simulink model "gm_LLE"  (R2020a)
settings: Solver=FixedStepDiscrete  StartTime=0.0  StopTime=T  FixedStep=1  RelTol=1e-3
InitFcn:
  | img_path = get_param('LLE/LowLightImage','FileName');
  | img = imread(img_path);
  | [m,n,c] = size(img);
  | 
  | h = [1, 2, 1; 2, 4, 2; 1, 2 ,1]./16;
  | h1 = flipud(fliplr(h));
  | T = (4000+(m+20)*(n+20));
undefined symbols (not defined in the file or in its folder): gray, m, n
libraries: visionfilter x10, visionhdlfilter x5, visionhdlio x4, visionhdlutilities x1, visionsources x1
settings Model: SimulationMode=accelerator  Creator=The MathWorks, Inc.  LastModifiedBy=25503
settings DataIOCC: ReturnWorkspaceOutputs=off
settings OptimizationCC: BlockReduction=off  ConditionallyExecuteInputs=off  DefaultParameterBehavior=Inlined
settings DebuggingCC: AlgebraicLoopMsg=error  InheritedTsInSrcMsg=none  ParameterPrecisionLossMsg=none  ArithmeticOperatorsInVariantConditions=warning
settings HardwareCC: ProdBitPerPointer=32  ProdBitPerSizeT=32  ProdBitPerPtrDiffT=32  ProdLargestAtomicFloat=None  ProdIntDivRoundTo=Undefined  ProdEndianess=Unspecified  ProdWordSize=32  ProdHWDeviceType=ASIC/FPGA->ASIC/FPGA  TargetBitPerPointer=64  TargetBitPerSizeT=64  TargetBitPerPtrDiffT=64  TargetLongLongMode=on  TargetIntDivRoundTo=Zero  TargetEndianess=LittleEndian  TargetWordSize=64  TargetHWDeviceType=Custom Processor->MATLAB Host Computer  ProdEqTarget=off
settings SFSimCC: SimUseLocalCustomCode=off  CustomCodeUndefinedFunction=UseInterfaceOnly
settings RTWCC: RTWUseLocalCustomCode=off

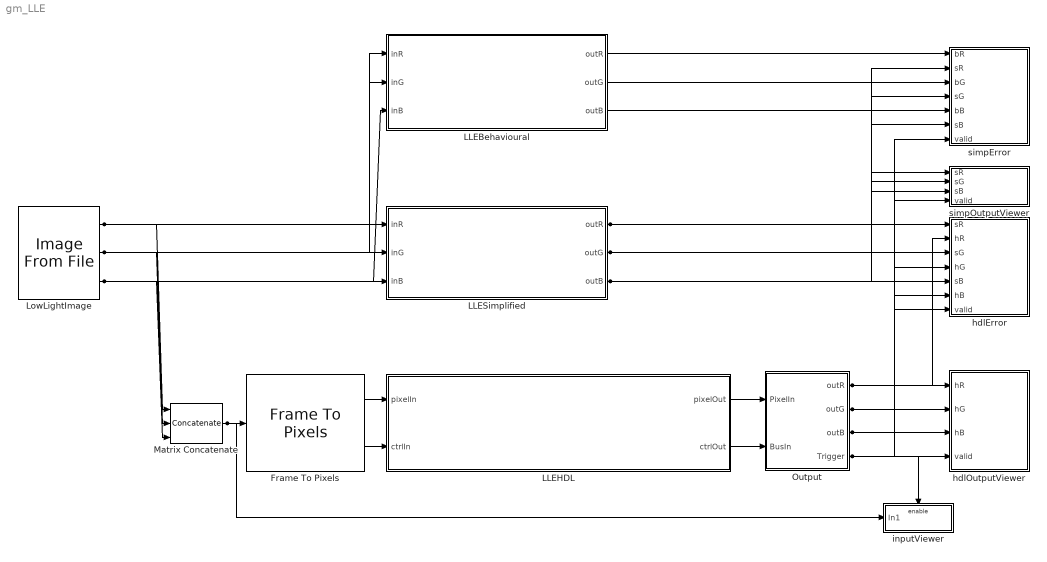
== system gm_LLE ==
  Frame To Pixels : visionhdlio/Frame To Pixels  NumComponents=c  NumPixels=1  VideoFormat=Custom  ActivePixelsPerLine=n  ActiveVideoLines=m  TotalPixelsPerLine=n+20  TotalVideoLines=m+20  StartingActiveLine=11  FrontPorch=10  SampleTime=0
      settings: SourceProductBaseCode=VT
  LLEBehavioural : Subsystem
  LLEHDL : Subsystem
  LLESimplified : Subsystem
  LowLightImage : visionsources/Image From File  Tag=vipblks_nd  FileName=C:\signal2\LLEHDL\myinput.jpg  Ts=(m+20)*(n+20)  imagePorts=Separate color signals  OutPortLabels=R|G|B  ImageDataType=Inherit from input image  sdImageDataType=uint(8)  Signed=on  WordLength=16  FractionLengthMode=User-defined  FractionLength=15
  Matrix Concatenate : Concatenate  NumInputs=3  Mode=Multidimensional array  ConcatenateDimension=3
  Output : Subsystem
  hdlError : Subsystem
  hdlOutputViewer : Subsystem
  inputViewer : Subsystem
  simpError : Subsystem
  simpOutputViewer : Subsystem
  wires:
  LLEBehavioural/2(outG) -> simpError/3(bG)
  LLEBehavioural/3(outB) -> simpError/5(bB)
  LLEBehavioural/1(outR) -> simpError/1(bR)
  LLESimplified/1(outR) -> hdlError/1(sR), simpOutputViewer/1(sR), simpError/2(sR)
  Matrix Concatenate/1 -> inputViewer/1(In1), Frame To Pixels/1
  Output/4(Trigger) -> inputViewer/Enable, hdlError/7(valid), simpOutputViewer/4(valid), simpError/7(valid), hdlOutputViewer/4(valid)
  LLESimplified/3(outB) -> hdlError/5(sB), simpOutputViewer/3(sB), simpError/6(sB)
  LLESimplified/2(outG) -> hdlError/3(sG), simpOutputViewer/2(sG), simpError/4(sG)
  Output/2(outG) -> hdlOutputViewer/2(hG), hdlError/4(hG)
  Output/1(outR) -> hdlError/2(hR), hdlOutputViewer/1(hR)
  Output/3(outB) -> hdlOutputViewer/3(hB), hdlError/6(hB)
  LowLightImage/3 -> Matrix Concatenate/3, LLEBehavioural/3(inB), LLESimplified/3(inB)
  LowLightImage/2 -> Matrix Concatenate/2, LLESimplified/2(inG), LLEBehavioural/2(inG)
  LowLightImage/1 -> Matrix Concatenate/1, LLEBehavioural/1(inR), LLESimplified/1(inR)
  LLEHDL/2(ctrlOut) -> Output/2(BusIn)
  LLEHDL/1(pixelOut) -> Output/1(PixelIn)
  Frame To Pixels/2 -> LLEHDL/2(ctrlIn)
  Frame To Pixels/1 -> LLEHDL/1(pixelIn)

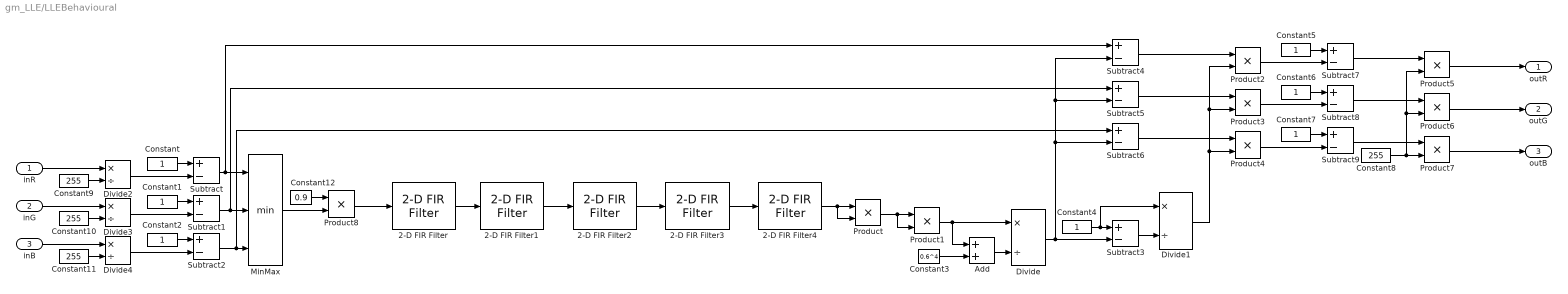
== system gm_LLE/LLEBehavioural ==
  inR : Inport
  inG : Inport  Port=2
  inB : Inport  Port=3
  2-D FIR Filter{,1..4} (5 alike) : visionfilter/2-D FIR Filter  separable=off  filtSrc=Specify via dialog  filterMtrx=h  verticalFilter=[4 0]  horizontalFilter=[4 0]  outSize=Same as input port I  padType=Replicate  padSrc=Specify via dialog  padVal=0  method=Convolution  firstCoeffMode=Binary point scaling  firstCoeffWordLength=16  firstCoeffFracLength=0  firstCoeffSignedness=Signed  firstCoeffLastDataTypeStr=fixdt(1,16,0)  outputSignedness=Auto  accumLastDataTypeStr=Inherit: Same as product output  roundingMode=Floor  overflowMode=off  firstCoeffDataTypeStr=fixdt(1,16,0)  firstCoeffMin=[]  firstCoeffMax=[]  accumDataTypeStr=Inherit: Same as product output  outputMin=[]  outputMax=[]
      settings: SourceProductBaseCode=VP
  Add : Sum
  Constant{,1..2,4..7} (7 alike) : Constant
  Constant10 : Constant  Value=255  OutDataTypeStr=double
  Constant11 : Constant  Value=255  OutDataTypeStr=double
  Constant12 : Constant  Value=0.9
  Constant3 : Constant  Value=0.6^4
  Constant8 : Constant  Value=255  OutDataTypeStr=uint8
  Constant9 : Constant  Value=255  OutDataTypeStr=double
  Divide{,1..4} (5 alike) : Product  Inputs=*/
  MinMax : MinMax  Inputs=3
  Product{,1..4,8} (6 alike) : Product
  Product5 : Product  OutDataTypeStr=uint8  RndMeth=Nearest  SaturateOnIntegerOverflow=on
  Product6 : Product  OutDataTypeStr=uint8  RndMeth=Nearest  SaturateOnIntegerOverflow=on
  Product7 : Product  OutDataTypeStr=uint8  RndMeth=Nearest  SaturateOnIntegerOverflow=on
  Subtract{,1..9} (10 alike) : Sum  Inputs=+-
  outR : Outport  VectorParamsAs1DForOutWhenUnconnected=off
  outG : Outport  Port=2  VectorParamsAs1DForOutWhenUnconnected=off
  outB : Outport  Port=3  VectorParamsAs1DForOutWhenUnconnected=off
  wires:
  Product7/1 -> outB/1
  inB/1 -> Divide4/1
  inG/1 -> Divide3/1
  Subtract5/1 -> Product3/1
  Constant12/1 -> Product8/1
  2-D FIR Filter3/1 -> 2-D FIR Filter4/1
  Constant5/1 -> Subtract7/1
  Product8/1 -> 2-D FIR Filter/1
  Constant6/1 -> Subtract8/1
  MinMax/1 -> Product8/2
  Subtract4/1 -> Product2/1
  Subtract9/1 -> Product7/1
  Product2/1 -> Subtract7/2
  Constant2/1 -> Subtract2/1
  Subtract8/1 -> Product6/1
  Constant8/1 -> Product5/2, Product6/2, Product7/2
  Product1/1 -> Divide/1, Add/1
  Subtract3/1 -> Divide1/2
  Product4/1 -> Subtract9/2
  Subtract2/1 -> MinMax/3, Subtract6/1
  Product6/1 -> outG/1
  Constant3/1 -> Add/2
  inR/1 -> Divide2/1
  Subtract6/1 -> Product4/1
  2-D FIR Filter1/1 -> 2-D FIR Filter2/1
  Subtract1/1 -> MinMax/2, Subtract5/1
  Constant4/1 -> Subtract3/1, Divide1/1
  Subtract7/1 -> Product5/1
  Product3/1 -> Subtract8/2
  Constant10/1 -> Divide3/2
  2-D FIR Filter/1 -> 2-D FIR Filter1/1
  2-D FIR Filter2/1 -> 2-D FIR Filter3/1
  Constant9/1 -> Divide2/2
  Subtract/1 -> MinMax/1, Subtract4/1
  Divide3/1 -> Subtract1/2
  Constant1/1 -> Subtract1/1
  Constant7/1 -> Subtract9/1
  Divide1/1 -> Product3/2, Product2/2, Product4/2
  Divide/1 -> Subtract3/2, Subtract6/2, Subtract4/2, Subtract5/2
  Constant11/1 -> Divide4/2
  Constant/1 -> Subtract/1
  Product/1 -> Product1/1, Product1/2
  Divide2/1 -> Subtract/2
  2-D FIR Filter4/1 -> Product/1, Product/2
  Divide4/1 -> Subtract2/2
  Add/1 -> Divide/2
  Product5/1 -> outR/1

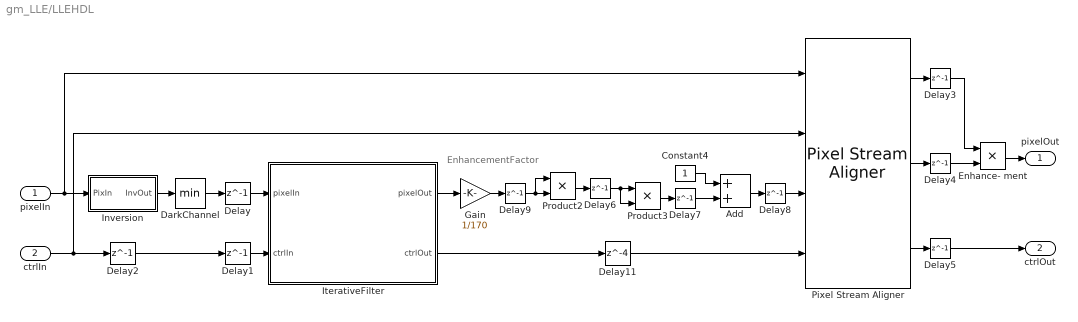
== system gm_LLE/LLEHDL ==
  note: EnhancementFactor
  pixelIn : Inport
  ctrlIn : Inport  Port=2
  Add : Sum  OutDataTypeStr=fixdt(0,30,22)  RndMeth=Nearest  SaturateOnIntegerOverflow=on
  Constant4 : Constant  OutDataTypeStr=fixdt(0,8,0)  SampleTime=-1
  DarkChannel : MinMax  RndMeth=Nearest  SaturateOnIntegerOverflow=on
  Delay{,1..9} (10 alike) : Delay  DelayLength=1
  Delay11 : Delay  DelayLength=4
  Enhance- ment : Product  OutDataTypeStr=uint8  RndMeth=Nearest  SaturateOnIntegerOverflow=on
  Gain : Gain  Gain=1/170  ParamDataTypeStr=fixdt(0,24,20)  OutDataTypeStr=fixdt(0,24,22)
  Inversion : Subsystem
  IterativeFilter : Subsystem
  Pixel Stream Aligner : visionhdlutilities/Pixel Stream Aligner  LineBufferSize=n  MaximumNumberOfLines=6  SimulateUsing=Code generation
      settings: SourceProductBaseCode=VT
  Product2 : Product  OutDataTypeStr=fixdt(0,26,22)  RndMeth=Nearest  SaturateOnIntegerOverflow=on
  Product3 : Product  OutDataTypeStr=fixdt(0,30,22)  RndMeth=Nearest  SaturateOnIntegerOverflow=on
  pixelOut : Outport  VectorParamsAs1DForOutWhenUnconnected=off
  ctrlOut : Outport  Port=2  VectorParamsAs1DForOutWhenUnconnected=off
  wires:
  IterativeFilter/2(ctrlOut) -> Delay11/1
  Delay9/1 -> Product2/2, Product2/1
  Delay5/1 -> ctrlOut/1
  Enhance- ment/1 -> pixelOut/1
  Delay11/1 -> Pixel Stream Aligner/4
  Delay8/1 -> Pixel Stream Aligner/3
  Gain/1 -> Delay9/1
  Delay/1 -> IterativeFilter/1(pixelIn)
  Delay1/1 -> IterativeFilter/2(ctrlIn)
  Add/1 -> Delay8/1
  Delay7/1 -> Add/2
  Delay6/1 -> Product3/1, Product3/2
  Constant4/1 -> Add/1
  Product3/1 -> Delay7/1
  Product2/1 -> Delay6/1
  IterativeFilter/1(pixelOut) -> Gain/1
  ctrlIn/1 -> Pixel Stream Aligner/2, Delay2/1
  Inversion/1(InvOut) -> DarkChannel/1
  Delay4/1 -> Enhance- ment/2
  Delay3/1 -> Enhance- ment/1
  Delay2/1 -> Delay1/1
  DarkChannel/1 -> Delay/1
  Pixel Stream Aligner/2 -> Delay4/1
  pixelIn/1 -> Pixel Stream Aligner/1, Inversion/1(PixIn)
  Pixel Stream Aligner/3 -> Delay5/1
  Pixel Stream Aligner/1 -> Delay3/1

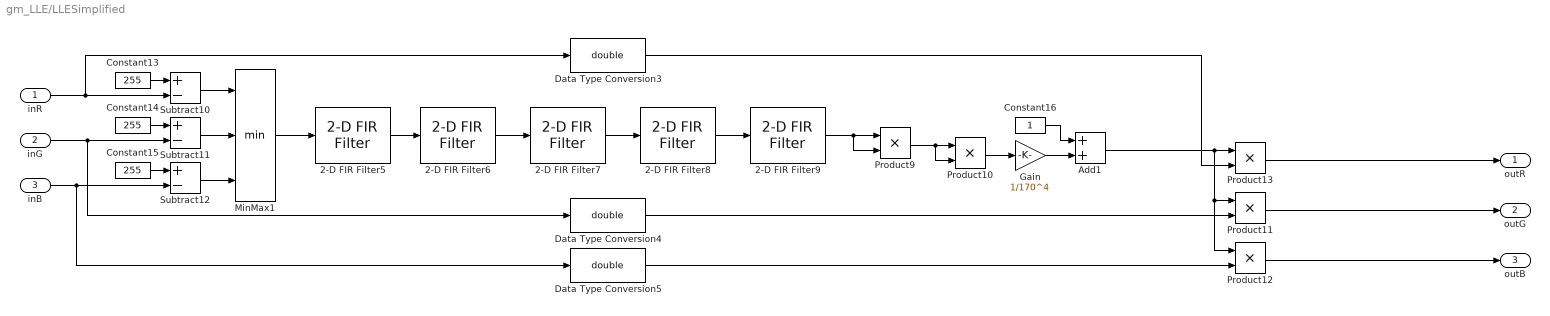
== system gm_LLE/LLESimplified ==
  inR : Inport
  inG : Inport  Port=2
  inB : Inport  Port=3
  2-D FIR Filter{5..9} (5 alike) : visionfilter/2-D FIR Filter  separable=off  filtSrc=Specify via dialog  filterMtrx=h  verticalFilter=[4 0]  horizontalFilter=[4 0]  outSize=Same as input port I  padType=Replicate  padSrc=Specify via dialog  padVal=0  method=Convolution  firstCoeffMode=Binary point scaling  firstCoeffWordLength=16  firstCoeffFracLength=0  firstCoeffSignedness=Signed  firstCoeffLastDataTypeStr=fixdt(1,16,0)  outputSignedness=Auto  accumLastDataTypeStr=Inherit: Same as product output  roundingMode=Floor  overflowMode=off  firstCoeffDataTypeStr=fixdt(1,16,0)  firstCoeffMin=[]  firstCoeffMax=[]  accumDataTypeStr=Inherit: Same as product output  outputMin=[]  outputMax=[]
      settings: SourceProductBaseCode=VP
  Add1 : Sum
  Constant13 : Constant  Value=255
  Constant14 : Constant  Value=255
  Constant15 : Constant  Value=255
  Constant16 : Constant
  Data Type Conversion3 : DataTypeConversion  OutDataTypeStr=double
  Data Type Conversion4 : DataTypeConversion  OutDataTypeStr=double
  Data Type Conversion5 : DataTypeConversion  OutDataTypeStr=double
  Gain : Gain  Gain=1/170^4
  MinMax1 : MinMax  Inputs=3
  Product10 : Product
  Product11 : Product  OutDataTypeStr=uint8  RndMeth=Nearest  SaturateOnIntegerOverflow=on
  Product12 : Product  OutDataTypeStr=uint8  RndMeth=Nearest  SaturateOnIntegerOverflow=on
  Product13 : Product  OutDataTypeStr=uint8  RndMeth=Nearest  SaturateOnIntegerOverflow=on
  Product9 : Product
  Subtract10 : Sum  Inputs=+-
  Subtract11 : Sum  Inputs=+-
  Subtract12 : Sum  Inputs=+-
  outR : Outport  VectorParamsAs1DForOutWhenUnconnected=off
  outG : Outport  Port=2  VectorParamsAs1DForOutWhenUnconnected=off
  outB : Outport  Port=3  VectorParamsAs1DForOutWhenUnconnected=off
  wires:
  Data Type Conversion5/1 -> Product12/2
  Data Type Conversion4/1 -> Product11/2
  Data Type Conversion3/1 -> Product13/2
  Product11/1 -> outG/1
  Product13/1 -> outR/1
  Constant13/1 -> Subtract10/1
  Constant16/1 -> Add1/1
  2-D FIR Filter9/1 -> Product9/2, Product9/1
  Constant14/1 -> Subtract11/1
  MinMax1/1 -> 2-D FIR Filter5/1
  Subtract10/1 -> MinMax1/1
  Add1/1 -> Product13/1, Product11/1, Product12/1
  2-D FIR Filter7/1 -> 2-D FIR Filter8/1
  2-D FIR Filter5/1 -> 2-D FIR Filter6/1
  Product9/1 -> Product10/1, Product10/2
  2-D FIR Filter6/1 -> 2-D FIR Filter7/1
  Product10/1 -> Gain/1
  inB/1 -> Subtract12/2, Data Type Conversion5/1
  Subtract12/1 -> MinMax1/3
  Gain/1 -> Add1/2
  inR/1 -> Subtract10/2, Data Type Conversion3/1
  Subtract11/1 -> MinMax1/2
  2-D FIR Filter8/1 -> 2-D FIR Filter9/1
  Product12/1 -> outB/1
  inG/1 -> Subtract11/2, Data Type Conversion4/1
  Constant15/1 -> Subtract12/1

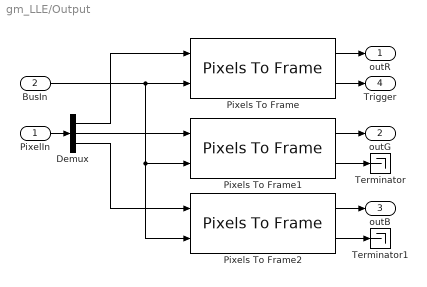
== system gm_LLE/Output ==
  PixelIn : Inport
  BusIn : Inport  Port=2
  Demux : Demux  Outputs=3
  Pixels To Frame : visionhdlio/Pixels To Frame  NumComponents=1  NumPixels=1  VideoFormat=Custom  ActivePixelsPerLine=n  ActiveVideoLines=m  TotalPixelsPerLine=n+20  TotalVideoLines=m+20
      settings: SourceProductBaseCode=VT
  Pixels To Frame1 : visionhdlio/Pixels To Frame  NumComponents=1  NumPixels=1  VideoFormat=Custom  ActivePixelsPerLine=n  ActiveVideoLines=m  TotalPixelsPerLine=n+20  TotalVideoLines=m+20
      settings: SourceProductBaseCode=VT
  Pixels To Frame2 : visionhdlio/Pixels To Frame  NumComponents=1  NumPixels=1  VideoFormat=Custom  ActivePixelsPerLine=n  ActiveVideoLines=m  TotalPixelsPerLine=n+20  TotalVideoLines=m+20
      settings: SourceProductBaseCode=VT
  Terminator : Terminator
  Terminator1 : Terminator
  outR : Outport  VectorParamsAs1DForOutWhenUnconnected=off
  outG : Outport  Port=2  VectorParamsAs1DForOutWhenUnconnected=off
  outB : Outport  Port=3  VectorParamsAs1DForOutWhenUnconnected=off
  Trigger : Outport  Port=4  VectorParamsAs1DForOutWhenUnconnected=off
  wires:
  Demux/1 -> Pixels To Frame/1
  PixelIn/1 -> Demux/1
  Pixels To Frame2/2 -> Terminator1/1
  BusIn/1 -> Pixels To Frame/2, Pixels To Frame1/2, Pixels To Frame2/2
  Demux/3 -> Pixels To Frame2/1
  Pixels To Frame2/1 -> outB/1
  Pixels To Frame1/2 -> Terminator/1
  Demux/2 -> Pixels To Frame1/1
  Pixels To Frame1/1 -> outG/1
  Pixels To Frame/2 -> Trigger/1
  Pixels To Frame/1 -> outR/1

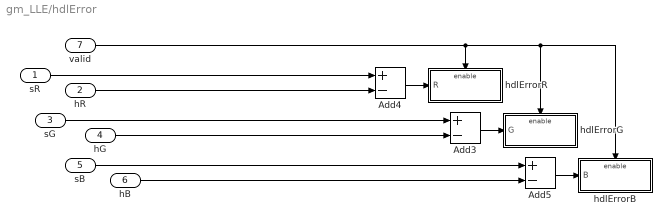
== system gm_LLE/hdlError ==
  sR : Inport
  hR : Inport  Port=2
  sG : Inport  Port=3
  hG : Inport  Port=4
  sB : Inport  Port=5
  hB : Inport  Port=6
  valid : Inport  Port=7
  Add3 : Sum  Inputs=+-  OutDataTypeStr=uint8  RndMeth=Nearest
  Add4 : Sum  Inputs=+-  OutDataTypeStr=uint8  RndMeth=Nearest
  Add5 : Sum  Inputs=+-  OutDataTypeStr=uint8  RndMeth=Nearest
  hdlErrorB : Subsystem
  hdlErrorG : Subsystem
  hdlErrorR : Subsystem
  wires:
  sR/1 -> Add4/1
  sB/1 -> Add5/1
  valid/1 -> hdlErrorR/Enable, hdlErrorG/Enable, hdlErrorB/Enable
  hG/1 -> Add3/2
  hR/1 -> Add4/2
  hB/1 -> Add5/2
  sG/1 -> Add3/1
  Add3/1 -> hdlErrorG/1(G)
  Add5/1 -> hdlErrorB/1(B)
  Add4/1 -> hdlErrorR/1(R)

== system gm_LLE/hdlOutputViewer ==
  hR : Inport
  hG : Inport  Port=2
  hB : Inport  Port=3
  valid : Inport  Port=4
  Matrix Concatenate1 : Concatenate  NumInputs=3  Mode=Multidimensional array  ConcatenateDimension=3
  hdlOutputViewer : Subsystem
  wires:
  valid/1 -> hdlOutputViewer/Enable
  hR/1 -> Matrix Concatenate1/1
  hB/1 -> Matrix Concatenate1/3
  hG/1 -> Matrix Concatenate1/2
  Matrix Concatenate1/1 -> hdlOutputViewer/1(In1)

== system gm_LLE/inputViewer ==
  In1 : Inport
  Enable : EnablePort
  LLEInput : VideoViewer  colormapValue=gray(256)  FigPos=[55.4 550.8 353.6 289.6]
  wires:
  In1/1 -> LLEInput/1

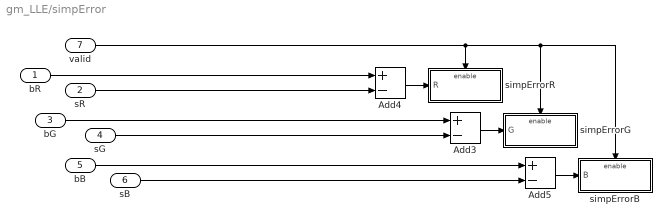
== system gm_LLE/simpError ==
  bR : Inport
  sR : Inport  Port=2
  bG : Inport  Port=3
  sG : Inport  Port=4
  bB : Inport  Port=5
  sB : Inport  Port=6
  valid : Inport  Port=7
  Add3 : Sum  Inputs=+-  OutDataTypeStr=uint8  RndMeth=Nearest
  Add4 : Sum  Inputs=+-  OutDataTypeStr=uint8  RndMeth=Nearest
  Add5 : Sum  Inputs=+-  OutDataTypeStr=uint8  RndMeth=Nearest
  simpErrorB : Subsystem
  simpErrorG : Subsystem
  simpErrorR : Subsystem
  wires:
  bR/1 -> Add4/1
  bB/1 -> Add5/1
  valid/1 -> simpErrorR/Enable, simpErrorG/Enable, simpErrorB/Enable
  sG/1 -> Add3/2
  sR/1 -> Add4/2
  sB/1 -> Add5/2
  bG/1 -> Add3/1
  Add3/1 -> simpErrorG/1(G)
  Add5/1 -> simpErrorB/1(B)
  Add4/1 -> simpErrorR/1(R)

== system gm_LLE/simpOutputViewer ==
  sR : Inport
  sG : Inport  Port=2
  sB : Inport  Port=3
  valid : Inport  Port=4
  Matrix Concatenate1 : Concatenate  NumInputs=3  Mode=Multidimensional array  ConcatenateDimension=3
  simpOutputViewer : Subsystem
  wires:
  valid/1 -> simpOutputViewer/Enable
  sR/1 -> Matrix Concatenate1/1
  sB/1 -> Matrix Concatenate1/3
  sG/1 -> Matrix Concatenate1/2
  Matrix Concatenate1/1 -> simpOutputViewer/1(In1)

== system gm_LLE/LLEHDL/Inversion ==
  PixIn : Inport
  Constant : Constant  Value=255  OutDataTypeStr=fixdt(0,8,0)  SampleTime=-1
  Delay : Delay  DelayLength=1
  Subtract : Sum  Inputs=+-  OutDataTypeStr=uint8  RndMeth=Nearest  SaturateOnIntegerOverflow=on
  InvOut : Outport  VectorParamsAs1DForOutWhenUnconnected=off
  wires:
  Delay/1 -> InvOut/1
  PixIn/1 -> Subtract/2
  Subtract/1 -> Delay/1
  Constant/1 -> Subtract/1

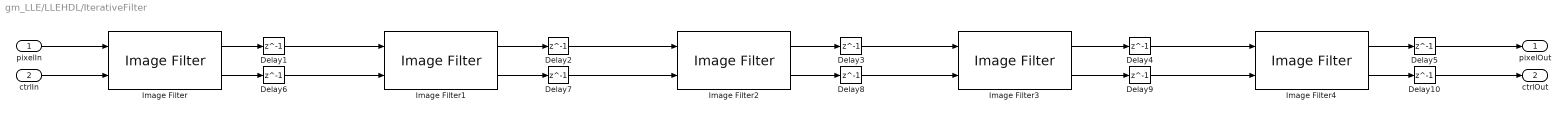
== system gm_LLE/LLEHDL/IterativeFilter ==
  pixelIn : Inport
  ctrlIn : Inport  Port=2
  Delay{1..10} (10 alike) : Delay  DelayLength=1
  Image Filter : visionhdlfilter/Image Filter  CoefficientsSource=Property  Coefficients=h1  PaddingMethod=Replicate  PaddingValue=0  LineBufferSize=2*n  SimulateUsing=Code generation  roundingMode=Nearest  overflowMode=on  CoeffDataTypeStr=fixdt(0,4,4)  CoeffMin=[]  CoeffMax=[]  OutputDataTypeStr=fixdt(0,12,4)  OutputMin=[]  OutputMax=[]
      settings: SourceProductBaseCode=VT
  Image Filter1 : visionhdlfilter/Image Filter  CoefficientsSource=Property  Coefficients=h1  PaddingMethod=Replicate  PaddingValue=0  LineBufferSize=2*n  SimulateUsing=Code generation  roundingMode=Nearest  overflowMode=on  CoeffDataTypeStr=fixdt(0,4,4)  CoeffMin=[]  CoeffMax=[]  OutputDataTypeStr=fixdt(0,16,8)  OutputMin=[]  OutputMax=[]
      settings: SourceProductBaseCode=VT
  Image Filter2 : visionhdlfilter/Image Filter  CoefficientsSource=Property  Coefficients=h1  PaddingMethod=Replicate  PaddingValue=0  LineBufferSize=2*n  SimulateUsing=Code generation  roundingMode=Nearest  overflowMode=on  CoeffDataTypeStr=fixdt(0,4,4)  CoeffMin=[]  CoeffMax=[]  OutputDataTypeStr=fixdt(0,20,12)  OutputMin=[]  OutputMax=[]
      settings: SourceProductBaseCode=VT
  Image Filter3 : visionhdlfilter/Image Filter  CoefficientsSource=Property  Coefficients=h1  PaddingMethod=Replicate  PaddingValue=0  LineBufferSize=2*n  SimulateUsing=Code generation  roundingMode=Nearest  overflowMode=on  CoeffDataTypeStr=fixdt(0,4,4)  CoeffMin=[]  CoeffMax=[]  OutputDataTypeStr=fixdt(0,24,16)  OutputMin=[]  OutputMax=[]
      settings: SourceProductBaseCode=VT
  Image Filter4 : visionhdlfilter/Image Filter  CoefficientsSource=Property  Coefficients=h1  PaddingMethod=Replicate  PaddingValue=0  LineBufferSize=2*n  SimulateUsing=Code generation  roundingMode=Nearest  overflowMode=on  CoeffDataTypeStr=fixdt(0,4,4)  CoeffMin=[]  CoeffMax=[]  OutputDataTypeStr=fixdt(0,28,20)  OutputMin=[]  OutputMax=[]
      settings: SourceProductBaseCode=VT
  pixelOut : Outport  VectorParamsAs1DForOutWhenUnconnected=off
  ctrlOut : Outport  Port=2  VectorParamsAs1DForOutWhenUnconnected=off
  wires:
  Delay10/1 -> ctrlOut/1
  Delay5/1 -> pixelOut/1
  Delay4/1 -> Image Filter4/1
  Delay9/1 -> Image Filter4/2
  Delay8/1 -> Image Filter3/2
  Delay3/1 -> Image Filter3/1
  Delay2/1 -> Image Filter2/1
  Delay7/1 -> Image Filter2/2
  Delay6/1 -> Image Filter1/2
  Delay1/1 -> Image Filter1/1
  Image Filter4/2 -> Delay10/1
  Image Filter4/1 -> Delay5/1
  Image Filter3/1 -> Delay4/1
  Image Filter2/1 -> Delay3/1
  Image Filter1/1 -> Delay2/1
  Image Filter/1 -> Delay1/1
  ctrlIn/1 -> Image Filter/2
  pixelIn/1 -> Image Filter/1
  Image Filter/2 -> Delay6/1
  Image Filter1/2 -> Delay7/1
  Image Filter2/2 -> Delay8/1
  Image Filter3/2 -> Delay9/1

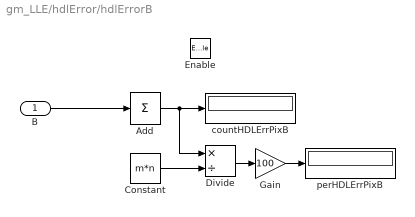
== system gm_LLE/hdlError/hdlErrorB ==
  B : Inport
  Enable : EnablePort
  Add : Sum  Inputs=+
  Constant : Constant  Value=m*n
  Divide : Product  Inputs=*/
  Gain : Gain  Gain=100
  countHDLErrPixB : Display
  perHDLErrPixB : Display
  wires:
  Divide/1 -> Gain/1
  Add/1 -> countHDLErrPixB/1, Divide/1
  Constant/1 -> Divide/2
  Gain/1 -> perHDLErrPixB/1
  B/1 -> Add/1

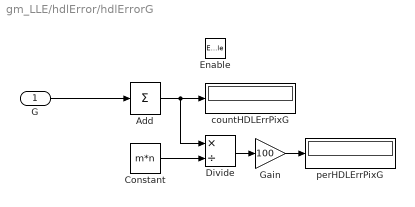
== system gm_LLE/hdlError/hdlErrorG ==
  G : Inport
  Enable : EnablePort
  Add : Sum  Inputs=+
  Constant : Constant  Value=m*n
  Divide : Product  Inputs=*/
  Gain : Gain  Gain=100
  countHDLErrPixG : Display
  perHDLErrPixG : Display
  wires:
  Gain/1 -> perHDLErrPixG/1
  Constant/1 -> Divide/2
  Add/1 -> countHDLErrPixG/1, Divide/1
  Divide/1 -> Gain/1
  G/1 -> Add/1

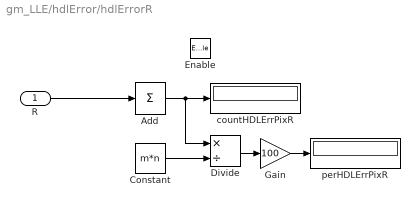
== system gm_LLE/hdlError/hdlErrorR ==
  R : Inport
  Enable : EnablePort
  Add : Sum  Inputs=+
  Constant : Constant  Value=m*n
  Divide : Product  Inputs=*/
  Gain : Gain  Gain=100
  countHDLErrPixR : Display
  perHDLErrPixR : Display
  wires:
  Gain/1 -> perHDLErrPixR/1
  Divide/1 -> Gain/1
  Constant/1 -> Divide/2
  Add/1 -> countHDLErrPixR/1, Divide/1
  R/1 -> Add/1

== system gm_LLE/hdlOutputViewer/hdlOutputViewer ==
  In1 : Inport
  Enable : EnablePort
  To Workspace : ToWorkspace  VariableName=lle_out  SampleTime=-1
      settings: Save2DSignal=2-D array (concatenate along first dimension)
  hdlLLEOutput : VideoViewer  colormapValue=gray(256)  FigPos=[781.8 550 352 290.4]
  wires:
  In1/1 -> To Workspace/1, hdlLLEOutput/1

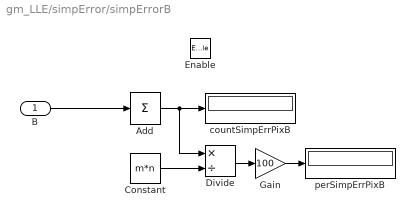
== system gm_LLE/simpError/simpErrorB ==
  B : Inport
  Enable : EnablePort
  Add : Sum  Inputs=+
  Constant : Constant  Value=m*n
  Divide : Product  Inputs=*/
  Gain : Gain  Gain=100
  countSimpErrPixB : Display
  perSimpErrPixB : Display
  wires:
  Divide/1 -> Gain/1
  Add/1 -> countSimpErrPixB/1, Divide/1
  Constant/1 -> Divide/2
  Gain/1 -> perSimpErrPixB/1
  B/1 -> Add/1

== system gm_LLE/simpError/simpErrorG ==
  G : Inport
  Enable : EnablePort
  Add : Sum  Inputs=+
  Constant : Constant  Value=m*n
  Divide : Product  Inputs=*/
  Gain : Gain  Gain=100
  countSimpErrPixG : Display
  perSimpErrPixG : Display
  wires:
  Gain/1 -> perSimpErrPixG/1
  Constant/1 -> Divide/2
  Add/1 -> countSimpErrPixG/1, Divide/1
  Divide/1 -> Gain/1
  G/1 -> Add/1

== system gm_LLE/simpError/simpErrorR ==
  R : Inport
  Enable : EnablePort
  Add : Sum  Inputs=+
  Constant : Constant  Value=m*n
  Divide : Product  Inputs=*/
  Gain : Gain  Gain=100
  countSimpErrPixR : Display
  perSimpErrPixR : Display
  wires:
  Gain/1 -> perSimpErrPixR/1
  Divide/1 -> Gain/1
  Constant/1 -> Divide/2
  Add/1 -> countSimpErrPixR/1, Divide/1
  R/1 -> Add/1

== system gm_LLE/simpOutputViewer/simpOutputViewer ==
  In1 : Inport
  Enable : EnablePort
  simpLLEOutput : VideoViewer  colormapValue=gray(256)  FigPos=[420.2 550.8 353.6 290.4]
  wires:
  In1/1 -> simpLLEOutput/1
